simulink model "zad2"  (R2020b)
settings: Solver=FixedStepDiscrete  StartTime=0.0  StopTime=0  RelTol=1e-3
libraries: CPOiS_SourcesSinks x9, CPOiS_HistogramOperations x3, CPOiS_DataManipulation x3, CPOiS_General x1
settings Model: Creator=jrybarz  LastModifiedBy=jrybarz

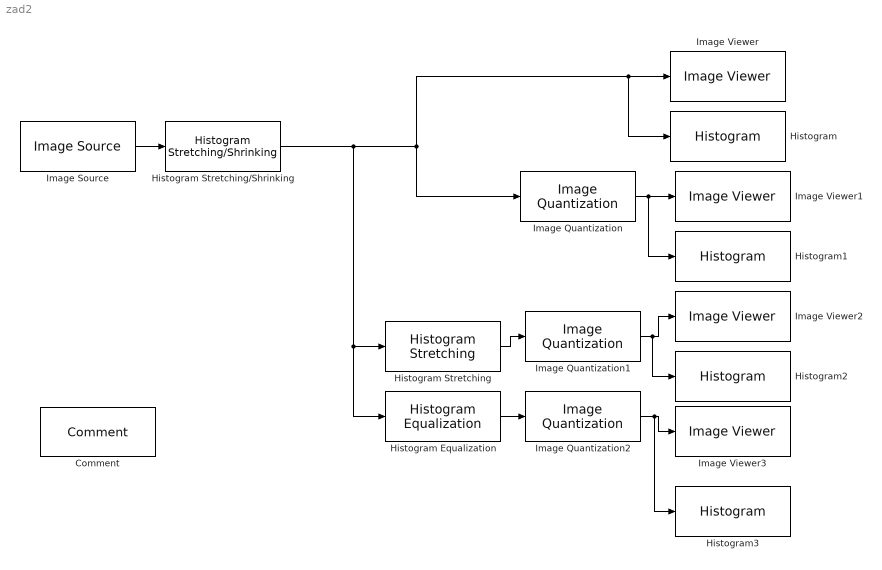
== system zad2 ==
  Comment : CPOiS_General/Comment
      settings: SourceProductName=CPOiS - Digital image and signal processing
  Histogram{,1..3} (4 alike) : CPOiS_SourcesSinks/Histogram
      settings: SourceProductName=CPOiS - Digital image and signal processing
  Histogram Stretching/Shrinking : CPOiS_HistogramOperations/Histogram Stretching//Shrinking  minimum=64  maximum=191
      settings: SourceProductName=CPOiS - Digital image and signal processing
  Histogram Equalization : CPOiS_HistogramOperations/Histogram Equalization
      settings: SourceProductName=CPOiS - Digital image and signal processing
  Histogram Stretching : CPOiS_HistogramOperations/Histogram Stretching
      settings: SourceProductName=CPOiS - Digital image and signal processing
  Image Quantization : CPOiS_DataManipulation/Image Quantization  LevelsNum=10
      settings: SourceProductName=CPOiS - Digital image and signal processing
  Image Quantization1 : CPOiS_DataManipulation/Image Quantization  LevelsNum=10
      settings: SourceProductName=CPOiS - Digital image and signal processing
  Image Quantization2 : CPOiS_DataManipulation/Image Quantization  LevelsNum=10
      settings: SourceProductName=CPOiS - Digital image and signal processing
  Image Source : CPOiS_SourcesSinks/Image Source  FileSelection=gull.png
      settings: SourceProductName=CPOiS - Digital image and signal processing
  Image Viewer{,1..3} (4 alike) : CPOiS_SourcesSinks/Image Viewer
      settings: SourceProductName=CPOiS - Digital image and signal processing
  wires:
  Image Source/1 -> Histogram Stretching/Shrinking/1
  Histogram Stretching/Shrinking/1 -> Histogram Equalization/1, Histogram Stretching/1, Image Quantization/1, Histogram/1, Image Viewer/1
  Image Quantization/1 -> Histogram1/1, Image Viewer1/1
  Image Quantization1/1 -> Histogram2/1, Image Viewer2/1
  Histogram Stretching/1 -> Image Quantization1/1
  Histogram Equalization/1 -> Image Quantization2/1
  Image Quantization2/1 -> Histogram3/1, Image Viewer3/1
